simulink model "base_rohrs_sigma_mod"  (R2025a)
settings: Solver=VariableStepAuto  StartTime=0.0  StopTime=100  RelTol=1e-3
libraries: simulink x1
settings Model: Creator=IHC  LastModifiedBy=sohrab
settings SolverCC: AlgebraicLoopSolver=TrustRegion
settings DebuggingCC: UnconnectedInputMsg=warning  UnconnectedOutputMsg=warning  UnconnectedLineMsg=warning  UnderSpecifiedDimensionMsg=warning
settings ModelReferenceCC: EnableRefExpFcnMdlSchedulingChecks=on
settings RTWCC: GPUComputeCapability=3.5

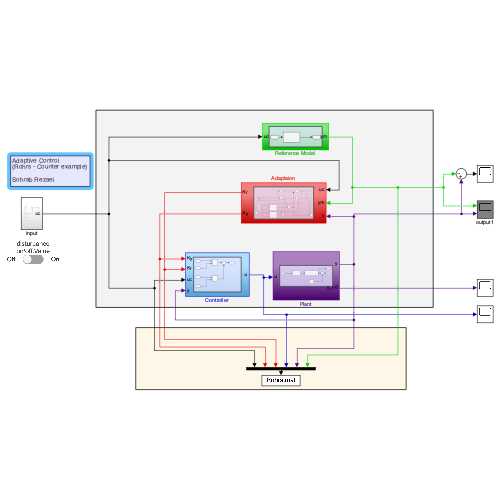
[thumbnail: Simulink's stored preview of the top-level diagram]
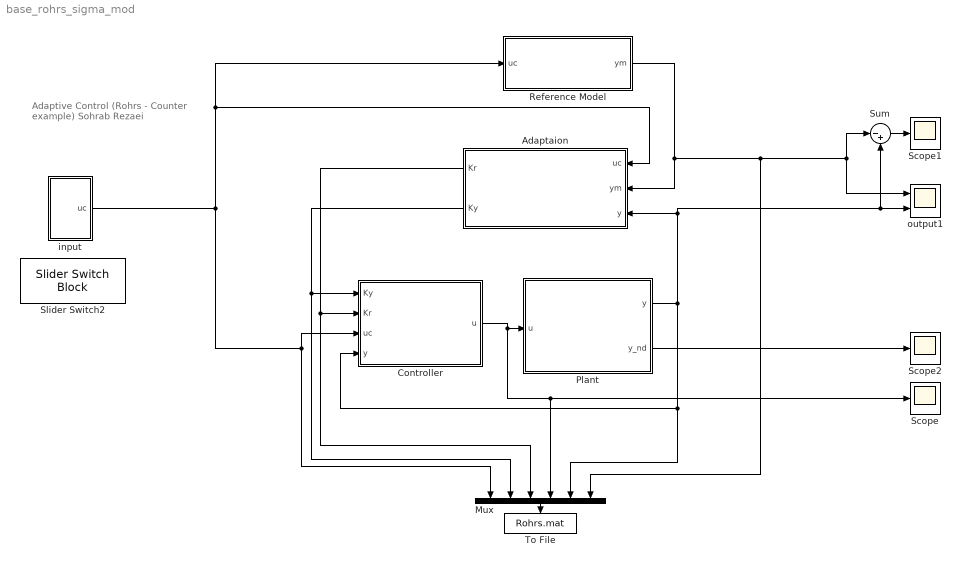
== system base_rohrs_sigma_mod ==
  note: Adaptive Control
      | (Rohrs - Counter example)
      |
      | Sohrab Rezaei
  Adaptaion : Subsystem
  Controller : Subsystem
  Mux : Mux  Inputs=6
  Plant : Subsystem
  Reference Model : Subsystem
  Scope : Scope
      settings: ActiveDisplayYMinimum=-0.89637  ActiveDisplayYMaximum=1.17674  DataLoggingVariableName=ScopeData2
  Scope1 : Scope
      settings: ActiveDisplayYMinimum=-0.16963  ActiveDisplayYMaximum=0.08827
  Scope2 : Scope
      settings: ActiveDisplayYMinimum=-0.55626  ActiveDisplayYMaximum=2.30162  DataLoggingVariableName=ScopeData2
  Slider Switch2 : SliderSwitchBlock
  Sum : Sum  Inputs=|-+
  To File : ToFile  Filename=Rohrs.mat  MatrixName=data
  input : Subsystem
  output1 : Scope  NumInputPorts=2
      settings: ActiveDisplayYMinimum=-0.05212  ActiveDisplayYMaximum=0.46909  DataLoggingVariableName=ScopeData3
  wires:
  Mux/1 -> To File/1
  input/1(uc) -> Reference Model/1(uc), Adaptaion/1(uc), Controller/3(uc), Mux/1
  Plant/1(y) -> Controller/4(y), Mux/5, output1/2, Sum/2, Adaptaion/3(y)
  Controller/1(u) -> Scope/1, Mux/4, Plant/1(u)
  Reference Model/1(ym) -> Mux/6, output1/1, Sum/1, Adaptaion/2(ym)
  Adaptaion/2(Ky) -> Mux/2, Controller/1(Ky)
  Adaptaion/1(Kr) -> Mux/3, Controller/2(Kr)
  Plant/2(y_nd) -> Scope2/1
  Sum/1 -> Scope1/1

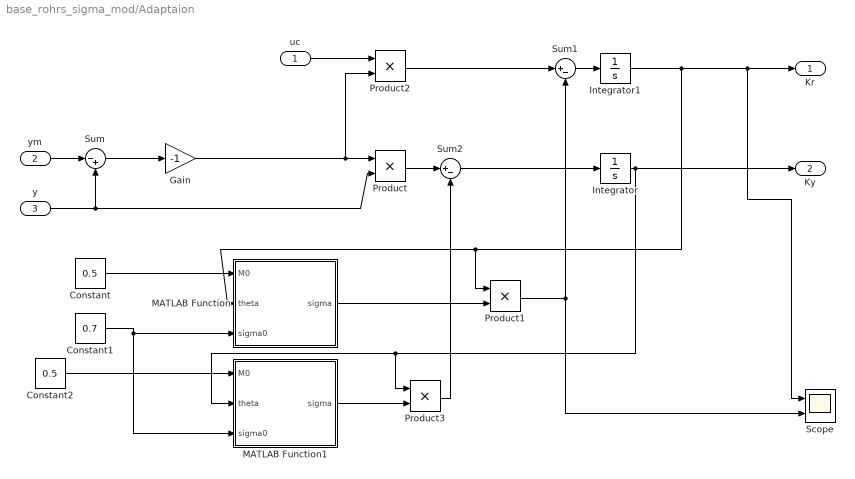
== system base_rohrs_sigma_mod/Adaptaion ==
  uc : Inport
  ym : Inport  Port=2
  y : Inport  Port=3
  Constant : Constant  Value=0.5
  Constant1 : Constant  Value=0.7
  Constant2 : Constant  Value=0.5
  Gain : Gain  Gain=-1
  Integrator : Integrator
  Integrator1 : Integrator
  MATLAB Function : MATLAB Function  TreatAsAtomicUnit=on
  MATLAB Function1 : MATLAB Function  TreatAsAtomicUnit=on
  Product{,1..3} (4 alike) : Product
  Scope : Scope  NumInputPorts=2
      settings: ActiveDisplayYMinimum=-0.07355  ActiveDisplayYMaximum=0.66192  DataLoggingVariableName=ScopeData3
  Sum : Sum  Inputs=|-+
  Sum1 : Sum  Inputs=|+-
  Sum2 : Sum  Inputs=|+-
  Kr : Outport
  Ky : Outport  Port=2
  wires:
  uc/1 -> Product2/1
  ym/1 -> Sum/1
  y/1 -> Product/2, Sum/2
  Sum/1 -> Gain/1
  Integrator/1 -> Product3/1, MATLAB Function1/2(theta), Ky/1
  Gain/1 -> Product2/2, Product/1
  Constant/1 -> MATLAB Function/1(M0)
  Constant1/1 -> MATLAB Function1/3(sigma0), MATLAB Function/3(sigma0)
  Sum1/1 -> Integrator1/1
  Product2/1 -> Sum1/1
  Sum2/1 -> Integrator/1
  Product/1 -> Sum2/1
  MATLAB Function1/1(sigma) -> Product3/2
  MATLAB Function/1(sigma) -> Product1/2
  Product1/1 -> Scope/2, Sum1/2
  Product3/1 -> Sum2/2
  Integrator1/1 -> Scope/1, Kr/1, Product1/1, MATLAB Function/2(theta)
  Constant2/1 -> MATLAB Function1/1(M0)

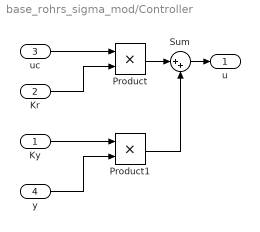
== system base_rohrs_sigma_mod/Controller ==
  Ky : Inport
  Kr : Inport  Port=2
  uc : Inport  Port=3
  y : Inport  Port=4
  Product : Product  RndMeth=Zero
  Product1 : Product  RndMeth=Zero
  Sum : Sum  Inputs=|++
  u : Outport
  wires:
  uc/1 -> Product/1
  Kr/1 -> Product/2
  Product/1 -> Sum/1
  Sum/1 -> u/1
  Ky/1 -> Product1/1
  y/1 -> Product1/2
  Product1/1 -> Sum/2

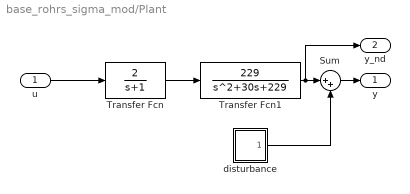
== system base_rohrs_sigma_mod/Plant ==
  u : Inport
  Sum : Sum  Inputs=|++
  Transfer Fcn : TransferFcn  Numerator=2  Denominator=[1 1]
  Transfer Fcn1 : TransferFcn  Numerator=229  Denominator=[1 30 229]
  disturbance : Subsystem
  y : Outport
  y_nd : Outport  Port=2
  wires:
  u/1 -> Transfer Fcn/1
  Transfer Fcn/1 -> Transfer Fcn1/1
  Transfer Fcn1/1 -> y_nd/1, Sum/1
  Sum/1 -> y/1
  disturbance/1(Out1) -> Sum/2

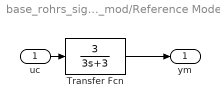
== system base_rohrs_sigma_mod/Reference Model ==
  uc : Inport
  Transfer Fcn : TransferFcn  Numerator=3  Denominator=[3 3]
  ym : Outport
  wires:
  uc/1 -> Transfer Fcn/1
  Transfer Fcn/1 -> ym/1

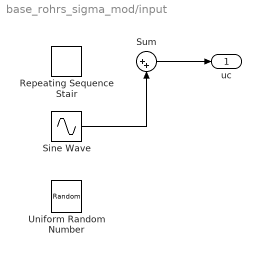
== system base_rohrs_sigma_mod/input ==
  Repeating Sequence Stair : simulink/Sources/Repeating Sequence Stair  OutValues="[3  4 1 ].'"  tsamp=60  OutMin=[]  OutMax=[]  OutDataTypeStr=double  OutputDataTypeScalingMode=double  OutDataType=fixdt(0,8)  ConRadixGroup=Best Precision: Vector-wise  OutScaling=2^-12
  Sine Wave : Sin  Amplitude=1.85  Bias=0.3  Frequency=16.1  SampleTime=0
  Sum : Sum  Inputs=|++
  Uniform Random Number : UniformRandomNumber  Minimum=-0.01  Maximum=0.01  SampleTime=0.1
  uc : Outport
  wires:
  Sum/1 -> uc/1
  Sine Wave/1 -> Sum/2

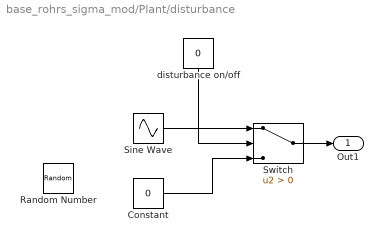
== system base_rohrs_sigma_mod/Plant/disturbance ==
  Constant : Constant  Value=0
  Random Number : RandomNumber  SampleTime=0.1
  Sine Wave : Sin  Amplitude=0.03  Frequency=10  SampleTime=0
  Switch : Switch  Criteria=u2 > Threshold  SaturateOnIntegerOverflow=off  InputSameDT=off
  disturbance on/off : Constant  Value=0
  Out1 : Outport
  wires:
  disturbance on/off/1 -> Switch/2
  Switch/1 -> Out1/1
  Constant/1 -> Switch/3
  Sine Wave/1 -> Switch/1

== matlab function base_rohrs_sigma_mod/Adaptaion/MATLAB Function ==
  data: M0 input; sigma output; theta input; sigma0 input
function sigma = fcn(M0,theta,sigma0)
tet=abs(theta);
tet=abs(theta);
    if tet<=M0
        sigma=0;

    elseif tet>M0 && tet<= 2*M0
        sigma=(tet/M0-1)*sigma0;

    else
        sigma=sigma0;
    end
end

== matlab function base_rohrs_sigma_mod/Adaptaion/MATLAB Function1 ==
  data: M0 input; sigma output; theta input; sigma0 input
function sigma = fcn(M0,theta,sigma0)
tet=abs(theta);
    if tet<=M0
        sigma=0;

    elseif tet>M0 && tet<= 2*M0
        sigma=(tet/M0-1)*sigma0;

    else
        sigma=sigma0;
    end
end
